simulink model "version_final_test 2"  (R2021b)
settings: Solver=VariableStepAuto  StartTime=0.0  StopTime=5  RelTol=1e-3
model workspace: external: MATLAB File D:\university\Semester 8\Intro to Robotics\Project\amali\Final_3\export second\Final_Assem_DataFile.m (data not in the file)
settings Model: Creator=admin  LastModifiedBy=ASUS

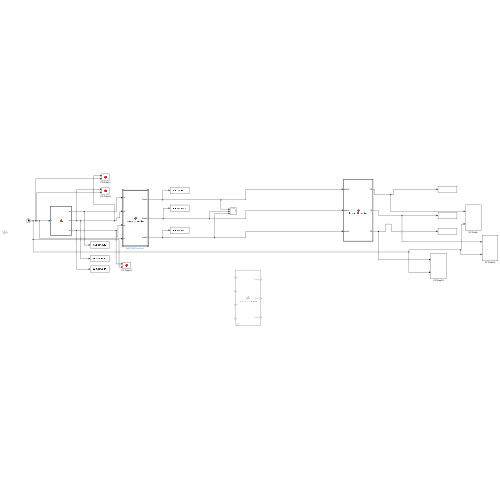
[thumbnail: Simulink's stored preview of the top-level diagram]
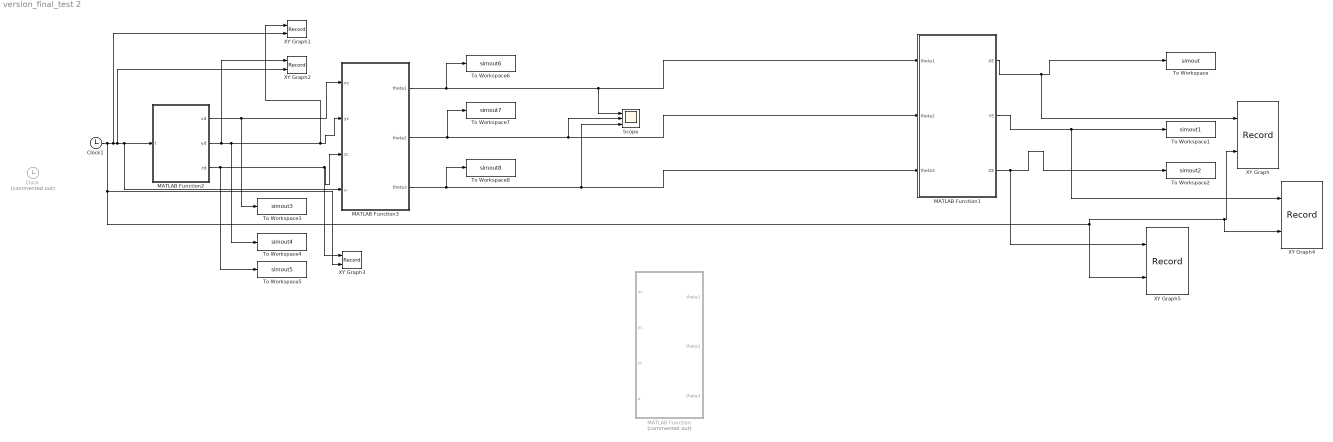
== system version_final_test 2 ==
  Clock : Clock  Commented=on
      settings: Decimation=u
  Clock1 : Clock
      settings: Decimation=tt
  MATLAB Function : MATLAB Function  Commented=on  TreatAsAtomicUnit=on
  MATLAB Function1 : MATLAB Function  TreatAsAtomicUnit=on
  MATLAB Function2 : MATLAB Function  TreatAsAtomicUnit=on
  MATLAB Function3 : MATLAB Function  TreatAsAtomicUnit=on
  Scope : Scope  NumInputPorts=3
  To Workspace : ToWorkspace  VariableName=simout  SampleTime=-1
      settings: Save2DSignal=2-D array (concatenate along first dimension)
  To Workspace1 : ToWorkspace  VariableName=simout1  SampleTime=-1
      settings: Save2DSignal=2-D array (concatenate along first dimension)
  To Workspace2 : ToWorkspace  VariableName=simout2  SampleTime=-1
      settings: Save2DSignal=2-D array (concatenate along first dimension)
  To Workspace3 : ToWorkspace  VariableName=simout3  SampleTime=-1
      settings: Save2DSignal=2-D array (concatenate along first dimension)
  To Workspace4 : ToWorkspace  VariableName=simout4  SampleTime=-1
      settings: Save2DSignal=2-D array (concatenate along first dimension)
  To Workspace5 : ToWorkspace  VariableName=simout5  SampleTime=-1
      settings: Save2DSignal=2-D array (concatenate along first dimension)
  To Workspace6 : ToWorkspace  VariableName=simout6  SaveFormat=Timeseries  SampleTime=-1
      settings: Save2DSignal=2-D array (concatenate along first dimension)
  To Workspace7 : ToWorkspace  VariableName=simout7  SaveFormat=Timeseries  SampleTime=-1
  To Workspace8 : ToWorkspace  VariableName=simout8  SaveFormat=Timeseries  SampleTime=-1
  XY Graph : Record  FileSettingsInternal="{\"entries\":[{\"content\":{\"excelSettings\":{\"content\":{},\"type\":\"Streamout.ExcelSettings\"}},\"type\":\"Streamout.FileSettingStorage\",\"uuid\":\"3e40fc56-9bf6-4325-82b9-e73c278979aa\"}],\"packageUris\":[\"http://schema.mathworks.com/mf0/streamout_blocks/R2020a\"],\"version\":\"1.0\"}"  Layout=[1 1]  SignalsInternal="{\"entries\":[{\"content\":{\"signals\":[{\"content\":{\"blockPath\":[\"sajad_version_final_test/XY Graph\"],\"channel\":[],\"dimensions\":[1],\"domain\":\"sajad_version_final_test/XY Graph\",\"lineColor\":\"#77ac30\",\"plots\":[],\"port\":1,\"sid\":[\"\"],\"signalID\":32769,\"signalName\":\"MATLAB Function1:1\"},\"type\":\"RecordBlkView.Signal\",\"uuid\":\"9c2c0287-0fe9-4151-84bc-b029ef1149d0\"},{\"content\":{\"blockPath\":[\"sajad_version_final_test/XY Graph\"],\"channel\":[],\"dimensions\":[1],\"domain\":\"sajad_version_final_test/XY Graph\",\"lineColor\":\"#4dbeee\",\"plots\":[],\"port\":2,\"sid\":[\"\"],\"signalID\":32773,\"signalName\":\"Clock1\"},\"type\":\"RecordBlkView.Signal\",\"uuid\":\"464b152c-b1b1-4cbe-9a9e-db401487d238\"}]},\"type\":\"RecordBlkView.InputSignals\",\"uuid\":\"5972ffab-4efb-4ac8-840a-e162470421a1\"}],\"packageUris\":[\"http://schema.mathworks.com/mf0/streamout_blocks/R2020a\"],\"version\":\"1.0\"}"  VisualizationBindings="{\"xyplotplugin\":{\"info\":[{\"series\":[],\"subplotID\":1}]}}"  CompatibilityTag=XY
  XY Graph1 : Record  FileSettingsInternal="{\"entries\":[{\"content\":{\"excelSettings\":{\"content\":{},\"type\":\"Streamout.ExcelSettings\"}},\"type\":\"Streamout.FileSettingStorage\",\"uuid\":\"532bc9f6-62b7-45a9-99ba-1d7b63b419cb\"}],\"packageUris\":[\"http://schema.mathworks.com/mf0/streamout_blocks/R2020a\"],\"version\":\"1.0\"}"  Layout=[1 1]  SignalsInternal="{\"entries\":[{\"content\":{\"signals\":[{\"content\":{\"blockPath\":[\"sajad_version_final_test/XY Graph1\"],\"channel\":[],\"dimensions\":[1],\"domain\":\"sajad_version_final_test/XY Graph1\",\"lineColor\":\"#a2142f\",\"plots\":[],\"port\":1,\"sid\":[\"\"],\"signalID\":32777,\"signalName\":\"MATLAB Function2:2\"},\"type\":\"RecordBlkView.Signal\",\"uuid\":\"b3da17f6-4959-4b1b-8f73-25e72f44b6ae\"},{\"content\":{\"blockPath\":[\"sajad_version_final_test/XY Graph1\"],\"channel\":[],\"dimensions\":[1],\"domain\":\"sajad_version_final_test/XY Graph1\",\"lineColor\":\"#139fff\",\"plots\":[],\"port\":2,\"sid\":[\"\"],\"signalID\":32781,\"signalName\":\"Clock1\"},\"type\":\"RecordBlkView.Signal\",\"uuid\":\"3861478f-2dcb-429f-94cb-a3b440a00b64\"}]},\"type\":\"RecordBlkView.InputSignals\",\"uuid\":\"b51e98e1-d9f2-4d33-b56f-c8a1df59121c\"}],\"packageUris\":[\"http://schema.mathworks.com/mf0/streamout_blocks/R2020a\"],\"version\":\"1.0\"}"  VisualizationBindings="{\"xyplotplugin\":{\"info\":[{\"series\":[],\"subplotID\":1}]}}"  CompatibilityTag=XY
  XY Graph2 : Record  FileSettingsInternal="{\"entries\":[{\"content\":{\"excelSettings\":{\"content\":{},\"type\":\"Streamout.ExcelSettings\"}},\"type\":\"Streamout.FileSettingStorage\",\"uuid\":\"936a8a69-01ec-4728-ac4d-0a2e35645a14\"}],\"packageUris\":[\"http://schema.mathworks.com/mf0/streamout_blocks/R2020a\"],\"version\":\"1.0\"}"  Layout=[1 1]  SignalsInternal="{\"entries\":[{\"content\":{\"signals\":[{\"content\":{\"blockPath\":[\"sajad_version_final_test/XY Graph2\"],\"channel\":[],\"dimensions\":[1],\"domain\":\"sajad_version_final_test/XY Graph2\",\"lineColor\":\"#ff6929\",\"plots\":[],\"port\":1,\"sid\":[\"\"],\"signalID\":32785,\"signalName\":\"MATLAB Function2:2\"},\"type\":\"RecordBlkView.Signal\",\"uuid\":\"50712de9-baee-4f43-8985-5ff43873bf88\"},{\"content\":{\"blockPath\":[\"sajad_version_final_test/XY Graph2\"],\"channel\":[],\"dimensions\":[1],\"domain\":\"sajad_version_final_test/XY Graph2\",\"lineColor\":\"#b746ff\",\"plots\":[],\"port\":2,\"sid\":[\"\"],\"signalID\":32789,\"signalName\":\"Clock1\"},\"type\":\"RecordBlkView.Signal\",\"uuid\":\"f8c7dc5f-f1b9-47ef-8695-d89aca68450c\"}]},\"type\":\"RecordBlkView.InputSignals\",\"uuid\":\"f720d26c-9fa6-439a-abe1-d60073326838\"}],\"packageUris\":[\"http://schema.mathworks.com/mf0/streamout_blocks/R2020a\"],\"version\":\"1.0\"}"  VisualizationBindings="{\"xyplotplugin\":{\"info\":[{\"series\":[],\"subplotID\":1}]}}"  CompatibilityTag=XY
  XY Graph3 : Record  FileSettingsInternal="{\"entries\":[{\"content\":{\"excelSettings\":{\"content\":{},\"type\":\"Streamout.ExcelSettings\"}},\"type\":\"Streamout.FileSettingStorage\",\"uuid\":\"ca2a5127-cc32-4c3a-b340-1d3aae6979dc\"}],\"packageUris\":[\"http://schema.mathworks.com/mf0/streamout_blocks/R2020a\"],\"version\":\"1.0\"}"  Layout=[1 1]  SignalsInternal="{\"entries\":[{\"content\":{\"signals\":[{\"content\":{\"blockPath\":[\"sajad_version_final_test/XY Graph3\"],\"channel\":[],\"dimensions\":[1],\"domain\":\"sajad_version_final_test/XY Graph3\",\"lineColor\":\"#64d413\",\"plots\":[],\"port\":1,\"sid\":[\"\"],\"signalID\":32793,\"signalName\":\"MATLAB Function2:3\"},\"type\":\"RecordBlkView.Signal\",\"uuid\":\"20780e5b-3c26-4332-97de-475beae32273\"},{\"content\":{\"blockPath\":[\"sajad_version_final_test/XY Graph3\"],\"channel\":[],\"dimensions\":[1],\"domain\":\"sajad_version_final_test/XY Graph3\",\"lineColor\":\"#ff13a6\",\"plots\":[],\"port\":2,\"sid\":[\"\"],\"signalID\":32797,\"signalName\":\"Clock1\"},\"type\":\"RecordBlkView.Signal\",\"uuid\":\"53bcd86c-a624-4f04-8711-e7424b38f953\"}]},\"type\":\"RecordBlkView.InputSignals\",\"uuid\":\"39be9750-27ac-4ba4-8e00-9be70ac9501f\"}],\"packageUris\":[\"http://schema.mathworks.com/mf0/streamout_blocks/R2020a\"],\"version\":\"1.0\"}"  VisualizationBindings="{\"xyplotplugin\":{\"info\":[{\"series\":[],\"subplotID\":1}]}}"  CompatibilityTag=XY
  XY Graph4 : Record  FileSettingsInternal="{\"entries\":[{\"content\":{\"excelSettings\":{\"content\":{},\"type\":\"Streamout.ExcelSettings\"}},\"type\":\"Streamout.FileSettingStorage\",\"uuid\":\"e5777caa-a0fe-45ac-b7cd-a0ba82adb5bb\"}],\"packageUris\":[\"http://schema.mathworks.com/mf0/streamout_blocks/R2020a\"],\"version\":\"1.0\"}"  Layout=[1 1]  SignalsInternal="{\"entries\":[{\"content\":{\"signals\":[{\"content\":{\"blockPath\":[\"sajad_version_final_test/XY Graph4\"],\"channel\":[],\"dimensions\":[1],\"domain\":\"sajad_version_final_test/XY Graph4\",\"lineColor\":\"#fe330a\",\"plots\":[],\"port\":1,\"sid\":[\"\"],\"signalID\":32801,\"signalName\":\"MATLAB Function1:2\"},\"type\":\"RecordBlkView.Signal\",\"uuid\":\"0b6e4854-ed0d-4476-8498-b0e0ba723788\"},{\"content\":{\"blockPath\":[\"sajad_version_final_test/XY Graph4\"],\"channel\":[],\"dimensions\":[1],\"domain\":\"sajad_version_final_test/XY Graph4\",\"lineColor\":\"#22b573\",\"plots\":[],\"port\":2,\"sid\":[\"\"],\"signalID\":32805,\"signalName\":\"Clock1\"},\"type\":\"RecordBlkView.Signal\",\"uuid\":\"1b74201d-6f60-4079-a22b-be1c548aac47\"}]},\"type\":\"RecordBlkView.InputSignals\",\"uuid\":\"3a69a391-6d08-4ec8-9a58-7bd51ddf57d8\"}],\"packageUris\":[\"http://schema.mathworks.com/mf0/streamout_blocks/R2020a\"],\"version\":\"1.0\"}"  VisualizationBindings="{\"xyplotplugin\":{\"info\":[{\"series\":[],\"subplotID\":1}]}}"  CompatibilityTag=XY
  XY Graph5 : Record  FileSettingsInternal="{\"entries\":[{\"content\":{\"excelSettings\":{\"content\":{},\"type\":\"Streamout.ExcelSettings\"}},\"type\":\"Streamout.FileSettingStorage\",\"uuid\":\"59ebff35-a092-4040-a83b-adeb36cc775f\"}],\"packageUris\":[\"http://schema.mathworks.com/mf0/streamout_blocks/R2020a\"],\"version\":\"1.0\"}"  Layout=[1 1]  SignalsInternal="{\"entries\":[{\"content\":{\"signals\":[{\"content\":{\"blockPath\":[\"sajad_version_final_test/XY Graph5\"],\"channel\":[],\"dimensions\":[1],\"domain\":\"sajad_version_final_test/XY Graph5\",\"lineColor\":\"#0072bd\",\"plots\":[],\"port\":1,\"sid\":[\"\"],\"signalID\":32809,\"signalName\":\"MATLAB Function1:3\"},\"type\":\"RecordBlkView.Signal\",\"uuid\":\"40184b4a-2e7b-4097-9eb7-859a7ed92f31\"},{\"content\":{\"blockPath\":[\"sajad_version_final_test/XY Graph5\"],\"channel\":[],\"dimensions\":[1],\"domain\":\"sajad_version_final_test/XY Graph5\",\"lineColor\":\"#d95319\",\"plots\":[],\"port\":2,\"sid\":[\"\"],\"signalID\":32813,\"signalName\":\"Clock1\"},\"type\":\"RecordBlkView.Signal\",\"uuid\":\"2f318857-8235-4a1c-9a65-a7053e9d47e0\"}]},\"type\":\"RecordBlkView.InputSignals\",\"uuid\":\"1fa74b36-d9f8-4c58-aeda-eab39448a368\"}],\"packageUris\":[\"http://schema.mathworks.com/mf0/streamout_blocks/R2020a\"],\"version\":\"1.0\"}"  VisualizationBindings="{\"xyplotplugin\":{\"info\":[{\"series\":[],\"subplotID\":1}]}}"  CompatibilityTag=XY
  wires:
  MATLAB Function2/1(xd) -> MATLAB Function3/1(xc), To Workspace3/1
  MATLAB Function2/2(yd) -> XY Graph2/1, To Workspace4/1, MATLAB Function3/2(yc), XY Graph1/1
  MATLAB Function2/3(zd) -> To Workspace5/1, MATLAB Function3/3(zc), XY Graph3/1
  MATLAB Function1/1(XE) -> XY Graph/1, To Workspace/1
  MATLAB Function1/2(YE) -> XY Graph4/1, To Workspace1/1
  MATLAB Function1/3(ZE) -> XY Graph5/1, To Workspace2/1
  Clock1/1 -> XY Graph3/2, XY Graph4/2, XY Graph/2, XY Graph5/2, XY Graph1/2, XY Graph2/2, MATLAB Function3/4(u), MATLAB Function2/1(t)
  MATLAB Function3/1(theta1) -> To Workspace6/1, Scope/1, MATLAB Function1/1(theta1)
  MATLAB Function3/2(theta2) -> To Workspace7/1, Scope/2, MATLAB Function1/2(theta2)
  MATLAB Function3/3(theta3) -> To Workspace8/1, Scope/3, MATLAB Function1/3(theta3)

== matlab function version_final_test 2/MATLAB Function1 ==
  data: theta1 input; XE output; theta2 input; theta3 input; YE output; ZE output
function [XE,YE,ZE]= forward_kinematics(theta1,theta2,theta3)
% 
% 
% xa= 0.224*cos(theta1)*sin(theta2) - 0.06821*cos(theta1) + 0.1*cos(theta1)*cos(theta2)*sin(theta3) + 0.1*cos(theta1)*cos(theta3)*sin(theta2);
% ya= 0.224*cos(theta1)*sin(theta2) - 0.06821*cos(theta1) + 0.1*cos(theta1)*cos(theta2)*sin(theta3) + 0.1*cos(theta1)*cos(theta3)*sin(theta2);
% za= 0.1*cos(theta2 + theta3) + 0.224*cos(theta2) + 0.178;

%a
a1=0;  %%% actualy a0
a2=-0.0165; %%% actualy a1
a3=0.217;   %%% L2   actualy a2
a4=0;     %%   actualy a3
%alpha
alphab1=  0;
alphab2= -pi/2;
alphab3=  0;
alphab4= -pi/2;
% d
d1 = 0.2867;
d2 = 0;
d3 = 0;
d4 = 0.1;  %%% L3
%theta
% theta2 = 0;
% theta3 = 0;
 theta4 =0;
T1=[cos(theta1) -sin(theta1) 0 a1;
   sin(theta1)*cos(alphab1) cos(theta1)*cos(alphab1) -sin(alphab1) -sin(alphab1)*d1;
   sin(theta1)*sin(alphab1) cos(theta1)*sin(alphab1) cos(alphab1) cos(alphab1)*d1;
   0 0 0 1];
T2=[cos(theta2) -sin(theta2) 0 a2;
   sin(theta2)*cos(alphab2) cos(theta2)*cos(alphab2) -sin(alphab2) -sin(alphab2)*d2;
   sin(theta2)*sin(alphab2) cos(theta2)*sin(alphab2) cos(alphab2) cos(alphab2)*d2;
   0 0 0 1];
T3=[cos(theta3) -sin(theta3) 0 a3;
   sin(theta3)*cos(alphab3) cos(theta3)*cos(alphab3) -sin(alphab3) -sin(alphab3)*d3;
   sin(theta3)*sin(alphab3) cos(theta3)*sin(alphab3) cos(alphab3) cos(alphab3)*d3;
   0 0 0 1];
 T4=[cos(theta4) -sin(theta4) 0 a4;
    sin(theta4)*cos(alphab4) cos(theta4)*cos(alphab4) -sin(alphab4) -sin(alphab4)*d4;
   sin(theta4)*sin(alphab4) cos(theta4)*sin(alphab4) cos(alphab4) cos(alphab4)*d4;
    0 0 0 1];
Ttotal = T1*T2*T3*T4;
XE = Ttotal(1,4);
YE = Ttotal(2,4);
ZE = Ttotal(3,4);

== matlab function version_final_test 2/MATLAB Function ==
  data: xc input; theta1 output; yc input; zc input; theta2 output; theta3 output; u input
function [theta1,theta2,theta3]= inverse_kinematics(xc,yc,zc,u)
theta1 = atan2(yc,xc)

xprim = (xc /cos(theta1))+ 0.0682;
yprim = (yc /sin(theta1))+0.0682;
zprim = zc - 0.178;
c_3 = (yprim^2+zprim^2-0.06)/(0.0449);
s_3 =(1-(1/2)*c_3^2);
theta3 = atan2(s_3,c_3)

c_2=((0.224*cos(theta1)+0.1*cos(theta3)*cos(theta1))*(zc-0.178))-(0.1*cos(theta3)*(xc+0.0682));
s_2=((xc+0.0682)*(0.1*sin(theta3)+0.224))-(zc-0.178)*(0.1*sin(theta3)*cos(theta1));
theta2 = atan2(s_2,c_2)
% d= 0.0165;
% d1= 0.196;
% a2= 0.217;
% a3=0.1;
% phi= atan2(xc,yc);
% r=sqrt(xc^2+yc^2);
% alpha= atan2(sqrt(r^2-d^2),d);
% theta1= phi- alpha
% s= zc-d1;
% rprim= sqrt(xc^2+yc^2-d^2);
% D= (rprim^2+s^2 - a2^2 - a3^2)/(2*a2*a3);
% if(u<5)
% theta3= atan2(D,sqrt(abs(1-D^2)))
% theta2=atan2(rprim,s)- atan2(a2 + a3*cos(theta3),a3*sin(theta3))
% else
% theta3= atan2(D,-sqrt(abs(1-D^2)));
% theta2=atan2(rprim,s)- atan2(a2 + a3*cos(theta3),a3*sin(theta3))
% end

== matlab function version_final_test 2/MATLAB Function2 ==
  data: t input; xd output; yd output; zd output
function [xd,yd,zd]=DT(t)

% xd= 0.2 - 0.2*sin((2*pi/5)*u + pi/2);
% yd= 0.3; %-1 - 0.5*cos((2*pi/5)*u + pi/2);
% zd= -0.5 - 0.5*cos((2*pi/5)*u + pi/2);
% if(t<5)
x0=0.1;  %0.15
y0=0.1;  %0.15
z0=0.5; %1
x1=-0.05; %-0.05
y1=0.05;  %0.05
z1=0.55; %2
s=t/5;
xd=x0+(x1-x0)*s; 
yd=y0+(y1-y0)*s;
zd=z0+(z1-z0)*s;
% else
% x0=0.05;
% y0=-0.05; %0.1
% z0=0.4;
% x1=0.1;
% y1=0.1;
% z1=0.15;
% s=(t-5)/5;
% xd=x0+(x1-x0)*s; 
% yd=y0+(y1-y0)*s;
% zd=z0+(z1-z0)*s;
% % v = (qi-qf)/(tb-tf)
end

== matlab function version_final_test 2/MATLAB Function3 ==
  data: xc input; theta1 output; yc input; zc input; theta2 output; theta3 output; u input
function [theta1,theta2,theta3]= inverse_kinematics(xc,yc,zc,u)
d= 0.0165;
% d1= 0.196;
d1 = 0.2867;
a2=-0.0165; %%% actualy a1
a3=0.217;   %%% L2   actualy a2
% a2= 0.217;
% a3=0.1;
phi= atan2(xc,yc);
r=sqrt(xc^2+yc^2);
alpha= atan2(sqrt(r^2-d^2),d);
theta1= phi- alpha;
s= zc-d1;
rprim= sqrt(xc^2+yc^2-d^2);
D= (rprim^2+s^2 - a2^2 - a3^2)/(2*a2*a3);
% if(u<5)
theta3= atan2(D,sqrt(abs(1-D^2)));
theta2=atan2(rprim,s)- atan2(a2 + a3*cos(theta3),a3*sin(theta3));
% else
% theta3= atan2(D,-sqrt(abs(1-D^2)));
% theta2=atan2(rprim,s)- atan2(a2 + a3*cos(theta3),a3*sin(theta3))
% end
